simulink model "rlOvertakeTwoCars"  (R2022b)
settings: Solver=ode45  StartTime=0.0  StopTime=inf  FixedStep=0.001  RelTol=5e-3
PreLoadFcn:
  | setUpModel
PostLoadFcn:
  | setUpMain
model workspace (MAT data in the model file):
  firstWarning = 0
  originalScenarioChecksum = 'F73A6DA3C723D3CA73A6F931B7A52A9C'
values from neighbouring files (symbols this model uses):
  accel_vec = (-4:0.5:4)'    [setUpModel.m]
  amax = 3    [setUpMain.m]
  amin = -3    [setUpMain.m]
  dyNorm = [dyNorm 1.1]    [setUpSlipstream.m]
  e1_initial = 0    [setUpMain.m]
  e2_initial = 0    [setUpMain.m]
  L = data.ActorSpecifications.Length    [setUpModel.m]
  psi_o1 = 0.0058 * (pi/180)    (= 0.000101229096616)    [setUpModel.m]
  psi_o2 = 0.3528 *(pi/180)    (= 0.00615752160104)    [setUpModel.m]
  ry = [ry 0]    [setUpSlipstream.m]
  ssSwitch = 1    [setUpSlipstream.m]
  tolpsi = 10 * pi/180    (= 0.174532925199)    [setUpSlipstream.m]
  toly = 1.2*W /2    [setUpSlipstream.m]
  Ts = 0.1    [setUpMPC.m]
  TsRL = Ts    [setUpRLEnv.m]
  umax = 0.3    [setUpMain.m]
  umin = -0.3    [setUpMain.m]
  v_o1 = highSpeed1    (= 35)    [setUpModel.m]
  v_o2 = highSpeed2    (= 36)    [setUpModel.m]
  vel1 = highSpeed1 * ones(length(xlt),length(ylt))    [setUpModel.m]
  vel2 = highSpeed2 * ones(length(xlt),length(ylt))    [setUpModel.m]
  vel_vec = 0:2:20    [setUpModel.m]
  W = data.ActorSpecifications(1,1).Width    [setUpSlipstream.m]
  X_o1 = xRef1(1)    [setUpModel.m]
  X_o2 = xRef2(1)    [setUpModel.m]
  xFollow = [0 x1 xFollow 60]    [setUpSlipstream.m]
  xLead = [0 -x0 xLead]    [setUpSlipstream.m]
  xlt = -250:10:200    [setUpModel.m]
  Y_o1 = yRef1(1)    [setUpModel.m]
  Y_o2 = yRef2(1)    [setUpModel.m]
  yFollow = [c y1 yFollow 1]    [setUpSlipstream.m]
  yLead = [c y0 yLead]    [setUpSlipstream.m]
  ylt = -150:10:100    [setUpModel.m]
undefined symbols (not defined in the file or in its folder): curvature1, curvature2, deg, DiscIntNeverNeededParam, gradbp1, gradbp2, psi, rad, s, v_o, x_colpen, x_o, y_colpen, Z_colpen
libraries: simulink x26, autolibsharedcommon x22, autolibutils x10, autolibshared x10, vehdynlibtirecommon x8, drivingscenarioandsensors x4, autolibpowerinfoutils x4, sharedtransform x4, aerolibconvert2 x2, simulink_extras x2, vehdynlibtire x2, mpcadaslib x1
(part 8 of 8)

== system rlOvertakeTwoCars/Vehicle Body 3DOF Dual Track Ego/Signal Routing/Signal Routing Dual/Lateral 3DOF/Hard Point Coordinate Transform Front Left ==
  InertFrmCg : Inport
  BdyFrmCg : Inport  Port=2
  Gain : Gain  Gain=-1/2
  Hard Point Coordinate Transform External Displacement : autolibsharedcommon/Hard Point Coordinate Transform External Displacement  aMode=aMode
  Selector : Selector  InputPortWidth=2  IndexOptions=Index vector (dialog)  Indices=[1]  OutputSizes=1
  Subtract : Sum  Inputs=+-
  Vector Concatenate : Concatenate  NumInputs=3
  a : Constant  Value=a
  d : Constant  Value=d
  h : Constant  Value=h
  w : Constant  Value=w
  Inert : Outport  VectorParamsAs1DForOutWhenUnconnected=off
  Body : Outport  Port=2  VectorParamsAs1DForOutWhenUnconnected=off
  wires:
  Subtract/1 -> Vector Concatenate/2
  d/1 -> Subtract/2
  InertFrmCg/1 -> Hard Point Coordinate Transform External Displacement/1
  w/1 -> Selector/1
  Gain/1 -> Subtract/1
  a/1 -> Vector Concatenate/1
  Hard Point Coordinate Transform External Displacement/2 -> Body/1
  Vector Concatenate/1 -> Hard Point Coordinate Transform External Displacement/3
  h/1 -> Vector Concatenate/3
  BdyFrmCg/1 -> Hard Point Coordinate Transform External Displacement/2
  Hard Point Coordinate Transform External Displacement/1 -> Inert/1
  Selector/1 -> Gain/1

== system rlOvertakeTwoCars/Vehicle Body 3DOF Dual Track Ego/Signal Routing/Signal Routing Dual/Lateral 3DOF/Hard Point Coordinate Transform Front Right ==
  InertFrmCg : Inport
  BdyFrmCg : Inport  Port=2
  Gain : Gain  Gain=1/2
  Hard Point Coordinate Transform External Displacement : autolibsharedcommon/Hard Point Coordinate Transform External Displacement  aMode=aMode
  Selector : Selector  InputPortWidth=2  IndexOptions=Index vector (dialog)  Indices=[1]  OutputSizes=1
  Subtract : Sum  Inputs=+-
  Vector Concatenate : Concatenate  NumInputs=3
  a : Constant  Value=a
  d : Constant  Value=d
  h : Constant  Value=h
  w : Constant  Value=w
  Inert : Outport  VectorParamsAs1DForOutWhenUnconnected=off
  Body : Outport  Port=2  VectorParamsAs1DForOutWhenUnconnected=off
  wires:
  Subtract/1 -> Vector Concatenate/2
  a/1 -> Vector Concatenate/1
  Selector/1 -> Gain/1
  h/1 -> Vector Concatenate/3
  w/1 -> Selector/1
  d/1 -> Subtract/2
  Gain/1 -> Subtract/1
  Hard Point Coordinate Transform External Displacement/1 -> Inert/1
  BdyFrmCg/1 -> Hard Point Coordinate Transform External Displacement/2
  Vector Concatenate/1 -> Hard Point Coordinate Transform External Displacement/3
  Hard Point Coordinate Transform External Displacement/2 -> Body/1
  InertFrmCg/1 -> Hard Point Coordinate Transform External Displacement/1

== system rlOvertakeTwoCars/Vehicle Body 3DOF Dual Track Ego/Signal Routing/Signal Routing Dual/Lateral 3DOF/Hard Point Coordinate Transform Geometric ==
  InertFrmCg : Inport
  BdyFrmCg : Inport  Port=2
  Hard Point Coordinate Transform External Displacement Beta : autolibsharedcommon/Hard Point Coordinate Transform External Displacement Beta  xdot_tol=xdot_tol  aMode=aMode
  Vector Concatenate : Concatenate  NumInputs=3
  latOff : Constant  Value=latOff
  longOff : Constant  Value=longOff
  vertOff : Constant  Value=vertOff
  Inert : Outport  VectorParamsAs1DForOutWhenUnconnected=off
  Body : Outport  Port=2  VectorParamsAs1DForOutWhenUnconnected=off
  wires:
  InertFrmCg/1 -> Hard Point Coordinate Transform External Displacement Beta/1
  Hard Point Coordinate Transform External Displacement Beta/2 -> Body/1
  Vector Concatenate/1 -> Hard Point Coordinate Transform External Displacement Beta/3
  BdyFrmCg/1 -> Hard Point Coordinate Transform External Displacement Beta/2
  Hard Point Coordinate Transform External Displacement Beta/1 -> Inert/1
  vertOff/1 -> Vector Concatenate/3
  longOff/1 -> Vector Concatenate/1
  latOff/1 -> Vector Concatenate/2

== system rlOvertakeTwoCars/Vehicle Body 3DOF Dual Track Ego/Signal Routing/Signal Routing Dual/Lateral 3DOF/Hard Point Coordinate Transform Rear Left ==
  InertFrmCg : Inport
  BdyFrmCg : Inport  Port=2
  Gain : Gain  Gain=-1/2
  Hard Point Coordinate Transform External Displacement : autolibsharedcommon/Hard Point Coordinate Transform External Displacement  aMode=aMode
  Selector : Selector  InputPortWidth=2  IndexOptions=Index vector (dialog)  Indices=[2]  OutputSizes=1
  Subtract : Sum  Inputs=+-
  Vector Concatenate : Concatenate  NumInputs=3
  b : Constant  Value=-b
  d : Constant  Value=d
  h : Constant  Value=h
  w : Constant  Value=w
  Inert : Outport  VectorParamsAs1DForOutWhenUnconnected=off
  Body : Outport  Port=2  VectorParamsAs1DForOutWhenUnconnected=off
  wires:
  Gain/1 -> Subtract/1
  Subtract/1 -> Vector Concatenate/2
  w/1 -> Selector/1
  d/1 -> Subtract/2
  Selector/1 -> Gain/1
  b/1 -> Vector Concatenate/1
  h/1 -> Vector Concatenate/3
  InertFrmCg/1 -> Hard Point Coordinate Transform External Displacement/1
  Hard Point Coordinate Transform External Displacement/2 -> Body/1
  Vector Concatenate/1 -> Hard Point Coordinate Transform External Displacement/3
  BdyFrmCg/1 -> Hard Point Coordinate Transform External Displacement/2
  Hard Point Coordinate Transform External Displacement/1 -> Inert/1

== system rlOvertakeTwoCars/Vehicle Body 3DOF Dual Track Ego/Signal Routing/Signal Routing Dual/Lateral 3DOF/Hard Point Coordinate Transform Rear Right ==
  InertFrmCg : Inport
  BdyFrmCg : Inport  Port=2
  Gain : Gain  Gain=1/2
  Hard Point Coordinate Transform External Displacement : autolibsharedcommon/Hard Point Coordinate Transform External Displacement  aMode=aMode
  Selector : Selector  InputPortWidth=2  IndexOptions=Index vector (dialog)  Indices=[2]  OutputSizes=1
  Subtract : Sum  Inputs=+-
  Vector Concatenate : Concatenate  NumInputs=3
  b : Constant  Value=-b
  d : Constant  Value=d
  h : Constant  Value=h
  w : Constant  Value=w
  Inert : Outport  VectorParamsAs1DForOutWhenUnconnected=off
  Body : Outport  Port=2  VectorParamsAs1DForOutWhenUnconnected=off
  wires:
  Gain/1 -> Subtract/1
  Subtract/1 -> Vector Concatenate/2
  w/1 -> Selector/1
  d/1 -> Subtract/2
  Selector/1 -> Gain/1
  b/1 -> Vector Concatenate/1
  h/1 -> Vector Concatenate/3
  Hard Point Coordinate Transform External Displacement/1 -> Inert/1
  BdyFrmCg/1 -> Hard Point Coordinate Transform External Displacement/2
  Vector Concatenate/1 -> Hard Point Coordinate Transform External Displacement/3
  Hard Point Coordinate Transform External Displacement/2 -> Body/1
  InertFrmCg/1 -> Hard Point Coordinate Transform External Displacement/1

== system rlOvertakeTwoCars/Vehicle Body 3DOF Dual Track Ego/Signal Routing/Signal Routing Dual/Lateral 3DOF/Hitch Coordinate Transform ==
  InertFrmCg : Inport
  BodyFrmCg : Inport  Port=2
  Constant : Constant  Value=dh
  Constant1 : Constant  Value=d
  Constant2 : Constant  Value=h
  Constant3 : Constant  Value=hh
  Constant4 : Constant  Value=hl
  Hard Point Coordinate Transform External Displacement : autolibsharedcommon/Hard Point Coordinate Transform External Displacement  aMode=aMode
  Sum : Sum  Inputs=|+-
  Sum1 : Sum  Inputs=|+-
  Unary Minus2 : UnaryMinus
  Vector Concatenate : Concatenate  NumInputs=3
  Inert : Outport
  Body : Outport  Port=2
  wires:
  Constant1/1 -> Sum1/2
  Unary Minus2/1 -> Vector Concatenate/1
  Constant/1 -> Unary Minus2/1
  Sum/1 -> Vector Concatenate/3
  Constant4/1 -> Sum1/1
  Sum1/1 -> Vector Concatenate/2
  Constant3/1 -> Sum/2
  Constant2/1 -> Sum/1
  BodyFrmCg/1 -> Hard Point Coordinate Transform External Displacement/2
  InertFrmCg/1 -> Hard Point Coordinate Transform External Displacement/1
  Vector Concatenate/1 -> Hard Point Coordinate Transform External Displacement/3
  Hard Point Coordinate Transform External Displacement/1 -> Inert/1
  Hard Point Coordinate Transform External Displacement/2 -> Body/1

== system rlOvertakeTwoCars/Vehicle Body 3DOF Dual Track Ego/Signal Routing/Signal Routing Dual/Power/xdot mode ==
  note: 1) Add Subsystem or Model blocks as valid variant choices.
      | 2) You cannot connect blocks at this level. At simulation, connectivity is automatically
      | determined, based on the active variant and port name matching.
  PFExt : Inport
  PMExt : Inport  Port=2
  PFh : Inport  Port=3
  PMh : Inport  Port=4
  PFDrag : Inport  Port=5
  PFwF : Inport  Port=6
  PFwR : Inport  Port=7
  BodyFrm : Inport  Port=8
  FxIn : Subsystem  VariantControl=1
  xdotin : Subsystem  VariantControl=0
  PF : Outport  VectorParamsAs1DForOutWhenUnconnected=off
  PM : Outport  Port=2  VectorParamsAs1DForOutWhenUnconnected=off
  ax : Outport  Port=3  VectorParamsAs1DForOutWhenUnconnected=off

== system rlOvertakeTwoCars/Vehicle Body 3DOF Dual Track/Signal Routing/Signal Routing/Power/xdot mode/FxIn ==
  PFExt : Inport
  PMExt : Inport  Port=2
  PFh : Inport  Port=3
  PMh : Inport  Port=4
  PFDrag : Inport  Port=5
  PFwF : Inport  Port=6
  PFwR : Inport  Port=7
  BodyFrm : Inport  Port=8
  Bus Selector2 : BusSelector  OutputSignals=Cg.Acc.ax
  Selector1 : Selector  InputPortWidth=3  IndexOptions=Index vector (dialog)  Indices=[1 2]  OutputSizes=1
  Selector2 : Selector  InputPortWidth=3  IndexOptions=Index vector (dialog)  Indices=[3]  OutputSizes=1
  Selector3 : Selector  InputPortWidth=3  IndexOptions=Index vector (dialog)  Indices=[3]  OutputSizes=1
  Selector4 : Selector  InputPortWidth=3  IndexOptions=Index vector (dialog)  Indices=[1 2]  OutputSizes=1
  Sum : Sum  Inputs=|++
  Sum1 : Sum  Inputs=|++
  Terminator : Terminator
  Terminator2 : Terminator
  Terminator3 : Terminator
  PF : Outport  VectorParamsAs1DForOutWhenUnconnected=off
  PM : Outport  Port=2  VectorParamsAs1DForOutWhenUnconnected=off
  ax : Outport  Port=3  VectorParamsAs1DForOutWhenUnconnected=off
  wires:
  Sum1/1 -> PF/1
  Selector4/1 -> Sum1/2
  PFh/1 -> Selector4/1
  Selector2/1 -> Sum/2
  Sum/1 -> PM/1
  PMh/1 -> Selector2/1
  PFExt/1 -> Selector1/1
  PMExt/1 -> Selector3/1
  PFDrag/1 -> Terminator/1
  Selector3/1 -> Sum/1
  Selector1/1 -> Sum1/1
  PFwR/1 -> Terminator3/1
  PFwF/1 -> Terminator2/1
  BodyFrm/1 -> Bus Selector2/1
  Bus Selector2/1 -> ax/1  "<ax>"

== system rlOvertakeTwoCars/Vehicle Body 3DOF Dual Track/Signal Routing/Signal Routing/Power/xdot mode/xdotin ==
  PFExt : Inport
  PMExt : Inport  Port=2
  PFh : Inport  Port=3
  PMh : Inport  Port=4
  PFDrag : Inport  Port=5
  PFwF : Inport  Port=6
  PFwR : Inport  Port=7
  BodyFrm : Inport  Port=8
  Add : Sum  Inputs=+++++
  Ground{,1..5} (6 alike) : Ground
  Mux{,1..4} (5 alike) : Mux  Inputs=2
  Selector1 : Selector  InputPortWidth=3  IndexOptions=Index vector (dialog)  Indices=[1]  OutputSizes=1
  Selector2 : Selector  InputPortWidth=3  IndexOptions=Index vector (dialog)  Indices=[2]  OutputSizes=1
  Selector3 : Selector  InputPortWidth=3  IndexOptions=Index vector (dialog)  Indices=[3]  OutputSizes=1
  Selector4 : Selector  InputPortWidth=3  IndexOptions=Index vector (dialog)  Indices=[1]  OutputSizes=1
  Selector5 : Selector  InputPortWidth=3  IndexOptions=Index vector (dialog)  Indices=[1]  OutputSizes=1
  Selector6 : Selector  InputPortWidth=3  IndexOptions=Index vector (dialog)  Indices=[2]  OutputSizes=1
  Selector7 : Selector  InputPortWidth=3  IndexOptions=Index vector (dialog)  Indices=[3]  OutputSizes=1
  Signal Specification : SignalSpecification  Unit=gn
  Sum : Sum  Inputs=|++
  Terminator : Terminator
  Unary Minus1 : UnaryMinus
  Unary Minus2 : UnaryMinus
  Unary Minus3 : UnaryMinus
  PF : Outport  VectorParamsAs1DForOutWhenUnconnected=off
  PM : Outport  Port=2  VectorParamsAs1DForOutWhenUnconnected=off
  ax : Outport  Port=3  VectorParamsAs1DForOutWhenUnconnected=off
  wires:
  Selector7/1 -> Sum/2
  Sum/1 -> PM/1
  PMh/1 -> Selector7/1
  PFh/1 -> Selector6/1
  Mux4/1 -> Add/4
  Ground5/1 -> Mux4/1
  Selector6/1 -> Mux4/2
  Add/1 -> PF/1
  PMExt/1 -> Selector3/1
  PFExt/1 -> Selector2/1
  PFDrag/1 -> Selector1/1
  Selector1/1 -> Unary Minus3/1
  Selector2/1 -> Mux/2
  Ground/1 -> Mux/1
  Mux/1 -> Add/3
  PFwF/1 -> Selector4/1
  PFwR/1 -> Selector5/1
  Ground1/1 -> Mux2/2
  Selector4/1 -> Unary Minus1/1
  Ground2/1 -> Mux1/2
  Selector5/1 -> Unary Minus2/1
  Mux2/1 -> Add/2
  Mux1/1 -> Add/1
  Unary Minus1/1 -> Mux1/1
  Unary Minus2/1 -> Mux2/1
  Ground3/1 -> Mux3/2
  Mux3/1 -> Add/5
  Selector3/1 -> Sum/1
  Unary Minus3/1 -> Mux3/1
  BodyFrm/1 -> Terminator/1
  Ground4/1 -> Signal Specification/1
  Signal Specification/1 -> ax/1

== system rlOvertakeTwoCars/Vehicle Body 3DOF Dual Track/Signal Routing/Signal Routing/state2bus/Angle Wrap/None ==
  u : Inport
  y : Outport  VectorParamsAs1DForOutWhenUnconnected=off
  wires:
  u/1 -> y/1

== system rlOvertakeTwoCars/Vehicle Body 3DOF Dual Track/Signal Routing/Signal Routing/state2bus/xddot2ax/m^22gn ==
  ay : Inport  Unit=m/s^2
  ax : Inport  Port=2  Unit=m/s^2
  Unit Conversion : UnitConversion
  Unit Conversion1 : UnitConversion
  ay_g : Outport  Unit=gn  VectorParamsAs1DForOutWhenUnconnected=off
  ax_g : Outport  Port=2  Unit=gn  VectorParamsAs1DForOutWhenUnconnected=off
  wires:
  Unit Conversion1/1 -> ax_g/1
  Unit Conversion/1 -> ay_g/1
  ax/1 -> Unit Conversion1/1
  ay/1 -> Unit Conversion/1

== system rlOvertakeTwoCars/Vehicle Body 3DOF Dual Track/Signal Routing/Signal Routing Dual/Power/xdot mode/FxIn ==
  PFExt : Inport
  PMExt : Inport  Port=2
  PFh : Inport  Port=3
  PMh : Inport  Port=4
  PFDrag : Inport  Port=5
  PFwF : Inport  Port=6
  PFwR : Inport  Port=7
  BodyFrm : Inport  Port=8
  Bus Selector2 : BusSelector  OutputSignals=Cg.Acc.ax
  Selector1 : Selector  InputPortWidth=3  IndexOptions=Index vector (dialog)  Indices=[1 2]  OutputSizes=1
  Selector2 : Selector  InputPortWidth=3  IndexOptions=Index vector (dialog)  Indices=[3]  OutputSizes=1
  Selector3 : Selector  InputPortWidth=3  IndexOptions=Index vector (dialog)  Indices=[3]  OutputSizes=1
  Selector4 : Selector  InputPortWidth=3  IndexOptions=Index vector (dialog)  Indices=[1 2]  OutputSizes=1
  Sum : Sum  Inputs=|++
  Sum1 : Sum  Inputs=|++
  Terminator : Terminator
  Terminator2 : Terminator
  Terminator3 : Terminator
  PF : Outport  VectorParamsAs1DForOutWhenUnconnected=off
  PM : Outport  Port=2  VectorParamsAs1DForOutWhenUnconnected=off
  ax : Outport  Port=3  VectorParamsAs1DForOutWhenUnconnected=off
  wires:
  Sum1/1 -> PF/1
  Selector4/1 -> Sum1/2
  PFh/1 -> Selector4/1
  Sum/1 -> PM/1
  Selector2/1 -> Sum/2
  PMh/1 -> Selector2/1
  PFExt/1 -> Selector1/1
  PMExt/1 -> Selector3/1
  PFDrag/1 -> Terminator/1
  Selector3/1 -> Sum/1
  Selector1/1 -> Sum1/1
  PFwR/1 -> Terminator3/1
  PFwF/1 -> Terminator2/1
  BodyFrm/1 -> Bus Selector2/1
  Bus Selector2/1 -> ax/1  "<ax>"

== system rlOvertakeTwoCars/Vehicle Body 3DOF Dual Track/Signal Routing/Signal Routing Dual/Power/xdot mode/xdotin ==
  PFExt : Inport
  PMExt : Inport  Port=2
  PFh : Inport  Port=3
  PMh : Inport  Port=4
  PFDrag : Inport  Port=5
  PFwF : Inport  Port=6
  PFwR : Inport  Port=7
  BodyFrm : Inport  Port=8
  Add : Sum  Inputs=+++++
  Ground{,1..5} (6 alike) : Ground
  Mux{,1..4} (5 alike) : Mux  Inputs=2
  Selector1 : Selector  InputPortWidth=3  IndexOptions=Index vector (dialog)  Indices=[1]  OutputSizes=1
  Selector2 : Selector  InputPortWidth=3  IndexOptions=Index vector (dialog)  Indices=[2]  OutputSizes=1
  Selector3 : Selector  InputPortWidth=3  IndexOptions=Index vector (dialog)  Indices=[3]  OutputSizes=1
  Selector4 : Selector  InputPortWidth=3  IndexOptions=Index vector (dialog)  Indices=[1]  OutputSizes=1
  Selector5 : Selector  InputPortWidth=3  IndexOptions=Index vector (dialog)  Indices=[1]  OutputSizes=1
  Selector6 : Selector  InputPortWidth=3  IndexOptions=Index vector (dialog)  Indices=[3]  OutputSizes=1
  Selector7 : Selector  InputPortWidth=3  IndexOptions=Index vector (dialog)  Indices=[2]  OutputSizes=1
  Signal Specification : SignalSpecification  Unit=gn
  Sum : Sum  Inputs=|++
  Terminator : Terminator
  Unary Minus1 : UnaryMinus
  Unary Minus2 : UnaryMinus
  Unary Minus3 : UnaryMinus
  PF : Outport  VectorParamsAs1DForOutWhenUnconnected=off
  PM : Outport  Port=2  VectorParamsAs1DForOutWhenUnconnected=off
  ax : Outport  Port=3  VectorParamsAs1DForOutWhenUnconnected=off
  wires:
  Mux4/1 -> Add/4
  Ground5/1 -> Mux4/1
  Selector7/1 -> Mux4/2
  PFh/1 -> Selector7/1
  Selector6/1 -> Sum/2
  Sum/1 -> PM/1
  PMh/1 -> Selector6/1
  Add/1 -> PF/1
  PMExt/1 -> Selector3/1
  PFExt/1 -> Selector2/1
  PFDrag/1 -> Selector1/1
  Selector1/1 -> Unary Minus3/1
  Selector2/1 -> Mux/2
  Ground/1 -> Mux/1
  Mux/1 -> Add/3
  PFwF/1 -> Selector4/1
  PFwR/1 -> Selector5/1
  Ground1/1 -> Mux2/2
  Selector4/1 -> Unary Minus1/1
  Ground2/1 -> Mux1/2
  Selector5/1 -> Unary Minus2/1
  Mux2/1 -> Add/2
  Mux1/1 -> Add/1
  Unary Minus1/1 -> Mux1/1
  Unary Minus2/1 -> Mux2/1
  Ground3/1 -> Mux3/2
  Mux3/1 -> Add/5
  Selector3/1 -> Sum/1
  Unary Minus3/1 -> Mux3/1
  BodyFrm/1 -> Terminator/1
  Ground4/1 -> Signal Specification/1
  Signal Specification/1 -> ax/1

== system rlOvertakeTwoCars/Vehicle Body 3DOF Dual Track Ego/Signal Routing/Signal Routing/Power/xdot mode/FxIn ==
  PFExt : Inport
  PMExt : Inport  Port=2
  PFh : Inport  Port=3
  PMh : Inport  Port=4
  PFDrag : Inport  Port=5
  PFwF : Inport  Port=6
  PFwR : Inport  Port=7
  BodyFrm : Inport  Port=8
  Bus Selector2 : BusSelector  OutputSignals=Cg.Acc.ax
  Selector1 : Selector  InputPortWidth=3  IndexOptions=Index vector (dialog)  Indices=[1 2]  OutputSizes=1
  Selector2 : Selector  InputPortWidth=3  IndexOptions=Index vector (dialog)  Indices=[3]  OutputSizes=1
  Selector3 : Selector  InputPortWidth=3  IndexOptions=Index vector (dialog)  Indices=[3]  OutputSizes=1
  Selector4 : Selector  InputPortWidth=3  IndexOptions=Index vector (dialog)  Indices=[1 2]  OutputSizes=1
  Sum : Sum  Inputs=|++
  Sum1 : Sum  Inputs=|++
  Terminator : Terminator
  Terminator2 : Terminator
  Terminator3 : Terminator
  PF : Outport  VectorParamsAs1DForOutWhenUnconnected=off
  PM : Outport  Port=2  VectorParamsAs1DForOutWhenUnconnected=off
  ax : Outport  Port=3  VectorParamsAs1DForOutWhenUnconnected=off
  wires:
  Sum1/1 -> PF/1
  Selector4/1 -> Sum1/2
  PFh/1 -> Selector4/1
  Selector2/1 -> Sum/2
  Sum/1 -> PM/1
  PMh/1 -> Selector2/1
  PFExt/1 -> Selector1/1
  PMExt/1 -> Selector3/1
  PFDrag/1 -> Terminator/1
  Selector3/1 -> Sum/1
  Selector1/1 -> Sum1/1
  PFwR/1 -> Terminator3/1
  PFwF/1 -> Terminator2/1
  BodyFrm/1 -> Bus Selector2/1
  Bus Selector2/1 -> ax/1  "<ax>"

== system rlOvertakeTwoCars/Vehicle Body 3DOF Dual Track Ego/Signal Routing/Signal Routing/Power/xdot mode/xdotin ==
  PFExt : Inport
  PMExt : Inport  Port=2
  PFh : Inport  Port=3
  PMh : Inport  Port=4
  PFDrag : Inport  Port=5
  PFwF : Inport  Port=6
  PFwR : Inport  Port=7
  BodyFrm : Inport  Port=8
  Add : Sum  Inputs=+++++
  Ground{,1..5} (6 alike) : Ground
  Mux{,1..4} (5 alike) : Mux  Inputs=2
  Selector1 : Selector  InputPortWidth=3  IndexOptions=Index vector (dialog)  Indices=[1]  OutputSizes=1
  Selector2 : Selector  InputPortWidth=3  IndexOptions=Index vector (dialog)  Indices=[2]  OutputSizes=1
  Selector3 : Selector  InputPortWidth=3  IndexOptions=Index vector (dialog)  Indices=[3]  OutputSizes=1
  Selector4 : Selector  InputPortWidth=3  IndexOptions=Index vector (dialog)  Indices=[1]  OutputSizes=1
  Selector5 : Selector  InputPortWidth=3  IndexOptions=Index vector (dialog)  Indices=[1]  OutputSizes=1
  Selector6 : Selector  InputPortWidth=3  IndexOptions=Index vector (dialog)  Indices=[2]  OutputSizes=1
  Selector7 : Selector  InputPortWidth=3  IndexOptions=Index vector (dialog)  Indices=[3]  OutputSizes=1
  Signal Specification : SignalSpecification  Unit=gn
  Sum : Sum  Inputs=|++
  Terminator : Terminator
  Unary Minus1 : UnaryMinus
  Unary Minus2 : UnaryMinus
  Unary Minus3 : UnaryMinus
  PF : Outport  VectorParamsAs1DForOutWhenUnconnected=off
  PM : Outport  Port=2  VectorParamsAs1DForOutWhenUnconnected=off
  ax : Outport  Port=3  VectorParamsAs1DForOutWhenUnconnected=off
  wires:
  Selector7/1 -> Sum/2
  Sum/1 -> PM/1
  PMh/1 -> Selector7/1
  PFh/1 -> Selector6/1
  Mux4/1 -> Add/4
  Ground5/1 -> Mux4/1
  Selector6/1 -> Mux4/2
  Add/1 -> PF/1
  PMExt/1 -> Selector3/1
  PFExt/1 -> Selector2/1
  PFDrag/1 -> Selector1/1
  Selector1/1 -> Unary Minus3/1
  Selector2/1 -> Mux/2
  Ground/1 -> Mux/1
  Mux/1 -> Add/3
  PFwF/1 -> Selector4/1
  PFwR/1 -> Selector5/1
  Ground1/1 -> Mux2/2
  Selector4/1 -> Unary Minus1/1
  Ground2/1 -> Mux1/2
  Selector5/1 -> Unary Minus2/1
  Mux2/1 -> Add/2
  Mux1/1 -> Add/1
  Unary Minus1/1 -> Mux1/1
  Unary Minus2/1 -> Mux2/1
  Ground3/1 -> Mux3/2
  Mux3/1 -> Add/5
  Selector3/1 -> Sum/1
  Unary Minus3/1 -> Mux3/1
  BodyFrm/1 -> Terminator/1
  Ground4/1 -> Signal Specification/1
  Signal Specification/1 -> ax/1

== system rlOvertakeTwoCars/Vehicle Body 3DOF Dual Track Ego/Signal Routing/Signal Routing/state2bus/Angle Wrap/None ==
  u : Inport
  y : Outport  VectorParamsAs1DForOutWhenUnconnected=off
  wires:
  u/1 -> y/1

== system rlOvertakeTwoCars/Vehicle Body 3DOF Dual Track Ego/Signal Routing/Signal Routing/state2bus/xddot2ax/m^22gn ==
  ay : Inport  Unit=m/s^2
  ax : Inport  Port=2  Unit=m/s^2
  Unit Conversion : UnitConversion
  Unit Conversion1 : UnitConversion
  ay_g : Outport  Unit=gn  VectorParamsAs1DForOutWhenUnconnected=off
  ax_g : Outport  Port=2  Unit=gn  VectorParamsAs1DForOutWhenUnconnected=off
  wires:
  Unit Conversion1/1 -> ax_g/1
  Unit Conversion/1 -> ay_g/1
  ax/1 -> Unit Conversion1/1
  ay/1 -> Unit Conversion/1

== system rlOvertakeTwoCars/Vehicle Body 3DOF Dual Track Ego/Signal Routing/Signal Routing Dual/Power/xdot mode/FxIn ==
  PFExt : Inport
  PMExt : Inport  Port=2
  PFh : Inport  Port=3
  PMh : Inport  Port=4
  PFDrag : Inport  Port=5
  PFwF : Inport  Port=6
  PFwR : Inport  Port=7
  BodyFrm : Inport  Port=8
  Bus Selector2 : BusSelector  OutputSignals=Cg.Acc.ax
  Selector1 : Selector  InputPortWidth=3  IndexOptions=Index vector (dialog)  Indices=[1 2]  OutputSizes=1
  Selector2 : Selector  InputPortWidth=3  IndexOptions=Index vector (dialog)  Indices=[3]  OutputSizes=1
  Selector3 : Selector  InputPortWidth=3  IndexOptions=Index vector (dialog)  Indices=[3]  OutputSizes=1
  Selector4 : Selector  InputPortWidth=3  IndexOptions=Index vector (dialog)  Indices=[1 2]  OutputSizes=1
  Sum : Sum  Inputs=|++
  Sum1 : Sum  Inputs=|++
  Terminator : Terminator
  Terminator2 : Terminator
  Terminator3 : Terminator
  PF : Outport  VectorParamsAs1DForOutWhenUnconnected=off
  PM : Outport  Port=2  VectorParamsAs1DForOutWhenUnconnected=off
  ax : Outport  Port=3  VectorParamsAs1DForOutWhenUnconnected=off
  wires:
  Sum1/1 -> PF/1
  Selector4/1 -> Sum1/2
  PFh/1 -> Selector4/1
  Sum/1 -> PM/1
  Selector2/1 -> Sum/2
  PMh/1 -> Selector2/1
  PFExt/1 -> Selector1/1
  PMExt/1 -> Selector3/1
  PFDrag/1 -> Terminator/1
  Selector3/1 -> Sum/1
  Selector1/1 -> Sum1/1
  PFwR/1 -> Terminator3/1
  PFwF/1 -> Terminator2/1
  BodyFrm/1 -> Bus Selector2/1
  Bus Selector2/1 -> ax/1  "<ax>"

== system rlOvertakeTwoCars/Vehicle Body 3DOF Dual Track Ego/Signal Routing/Signal Routing Dual/Power/xdot mode/xdotin ==
  PFExt : Inport
  PMExt : Inport  Port=2
  PFh : Inport  Port=3
  PMh : Inport  Port=4
  PFDrag : Inport  Port=5
  PFwF : Inport  Port=6
  PFwR : Inport  Port=7
  BodyFrm : Inport  Port=8
  Add : Sum  Inputs=+++++
  Ground{,1..5} (6 alike) : Ground
  Mux{,1..4} (5 alike) : Mux  Inputs=2
  Selector1 : Selector  InputPortWidth=3  IndexOptions=Index vector (dialog)  Indices=[1]  OutputSizes=1
  Selector2 : Selector  InputPortWidth=3  IndexOptions=Index vector (dialog)  Indices=[2]  OutputSizes=1
  Selector3 : Selector  InputPortWidth=3  IndexOptions=Index vector (dialog)  Indices=[3]  OutputSizes=1
  Selector4 : Selector  InputPortWidth=3  IndexOptions=Index vector (dialog)  Indices=[1]  OutputSizes=1
  Selector5 : Selector  InputPortWidth=3  IndexOptions=Index vector (dialog)  Indices=[1]  OutputSizes=1
  Selector6 : Selector  InputPortWidth=3  IndexOptions=Index vector (dialog)  Indices=[3]  OutputSizes=1
  Selector7 : Selector  InputPortWidth=3  IndexOptions=Index vector (dialog)  Indices=[2]  OutputSizes=1
  Signal Specification : SignalSpecification  Unit=gn
  Sum : Sum  Inputs=|++
  Terminator : Terminator
  Unary Minus1 : UnaryMinus
  Unary Minus2 : UnaryMinus
  Unary Minus3 : UnaryMinus
  PF : Outport  VectorParamsAs1DForOutWhenUnconnected=off
  PM : Outport  Port=2  VectorParamsAs1DForOutWhenUnconnected=off
  ax : Outport  Port=3  VectorParamsAs1DForOutWhenUnconnected=off
  wires:
  Mux4/1 -> Add/4
  Ground5/1 -> Mux4/1
  Selector7/1 -> Mux4/2
  PFh/1 -> Selector7/1
  Selector6/1 -> Sum/2
  Sum/1 -> PM/1
  PMh/1 -> Selector6/1
  Add/1 -> PF/1
  PMExt/1 -> Selector3/1
  PFExt/1 -> Selector2/1
  PFDrag/1 -> Selector1/1
  Selector1/1 -> Unary Minus3/1
  Selector2/1 -> Mux/2
  Ground/1 -> Mux/1
  Mux/1 -> Add/3
  PFwF/1 -> Selector4/1
  PFwR/1 -> Selector5/1
  Ground1/1 -> Mux2/2
  Selector4/1 -> Unary Minus1/1
  Ground2/1 -> Mux1/2
  Selector5/1 -> Unary Minus2/1
  Mux2/1 -> Add/2
  Mux1/1 -> Add/1
  Unary Minus1/1 -> Mux1/1
  Unary Minus2/1 -> Mux2/1
  Ground3/1 -> Mux3/2
  Mux3/1 -> Add/5
  Selector3/1 -> Sum/1
  Unary Minus3/1 -> Mux3/1
  BodyFrm/1 -> Terminator/1
  Ground4/1 -> Signal Specification/1
  Signal Specification/1 -> ax/1

== matlab function rlOvertakeTwoCars/Vehicle Body 3DOF Dual Track Ego/Signal Routing/Signal Routing/state2bus/COMB2I ==
  data: x input size=4; y output size=2
function y = fcn(x)%#codegen
coder.allowpcode('plain')
y = automlvehb2i(x);

== matlab function rlOvertakeTwoCars/Final Trajectory Bird's-Eye Visualization Lead/MATLAB Function ==
  data: pos input; egoActor output Bus: BusActorsActors; vel input; yaw input; yawRate input
function egoActor = packEgo(pos,vel,yaw,yawRate)
% Pack ego information into a single ego actor bus
%
% Imoprtant note:
% Output is a bus of type BusActorsActors. This is the same bus used by the
% Scenario Reader to output an individual actor. If you change the
% output bus name of Scenario Reader, change the output bus name here
% as well by clicking on 'Edit Data' in the menu above.

egoActor = struct(...
    'ActorID',1,...
    'Position', [pos(1) pos(2) 0], ...
    'Velocity', [vel(1) vel(2) 0], ...
    'Roll', 0, ...
    'Pitch', 0, ...
    'Yaw', yaw, ...
    'AngularVelocity', [0 0 yawRate]);

== matlab function rlOvertakeTwoCars/Vehicle Body 3DOF Dual Track Ego/Signal Routing/Signal Routing Dual/state2bus/COMB2I ==
  data: x input size=4; y output size=2
function y = fcn(x)%#codegen
coder.allowpcode('plain')
y = automlvehb2i(x);

== matlab function rlOvertakeTwoCars/Vehicle Body 3DOF Dual Track Ego/vehicle model ==
  data: delta_f input; delta_r input; mu input; a parameter; b parameter; h parameter; d parameter; w parameter; m parameter; NF parameter; NR parameter; Izz parameter; g parameter; Fxtire_sat parameter size=1; Fytire_sat parameter size=1; trackMode parameter; inputMode parameter; xdot_tol parameter; Fznom parameter size=1; F_f input; F_r input; F_ext input size=3; M_ext input size=3; Fh input size=3; Mh input size=3; Cy_f input; Cy_r input; dh input; hl input; hh input; yOut output size=3; FBody output size=3; MBody output size=3; FOut output; FTire output; Fg output size=3; wheelInfo output; stateDer output size=4; stateVec input size=4; status output size=1
function [yOut,FBody,MBody,FOut,FTire,Fg,wheelInfo,stateDer,status] = fcn(delta_f,delta_r,mu,a,b,h,d,w,m,NF,NR,Izz,g,Fxtire_sat,Fytire_sat,trackMode,inputMode,xdot_tol,Fznom,F_f,F_r,F_ext,M_ext,Fh,Mh,Cy_f,Cy_r,dh,hl,hh,stateVec)%#codegen
coder.allowpcode('plain')
switch trackMode
    case 1
       [yOut,FBody,MBody,FOut,FTire,Fg,wheelInfo,stateDer,status] = automlvehdynbicycle(delta_f,delta_r,mu,a,b,h,m,NF,NR,Izz,g,Fxtire_sat,Fytire_sat,inputMode,xdot_tol,Fznom,F_f,F_r,F_ext,M_ext,Fh,Mh,Cy_f,Cy_r,dh,hh,stateVec);
    case 2
       [yOut,FBody,MBody,FOut,FTire,Fg,wheelInfo,stateDer,status] = automlvehdyndualtrack(delta_f,delta_r,mu,a,b,h,d,w,m,NF,NR,Izz,g,Fxtire_sat,Fytire_sat,inputMode,xdot_tol,Fznom,F_f,F_r,F_ext,M_ext,Fh,Mh,Cy_f,Cy_r,dh,hl,hh,stateVec);
end
end

== matlab function rlOvertakeTwoCars/Final Trajectory Bird's-Eye Visualization Ego/MATLAB Function ==
  data: pos input; egoActor output Bus: BusActorsActors; vel input; yaw input; yawRate input
function egoActor = packEgo(pos,vel,yaw,yawRate)
% Pack ego information into a single ego actor bus
%
% Imoprtant note:
% Output is a bus of type BusActorsActors. This is the same bus used by the
% Scenario Reader to output an individual actor. If you change the
% output bus name of Scenario Reader, change the output bus name here
% as well by clicking on 'Edit Data' in the menu above.

egoActor = struct(...
    'ActorID',2,...
    'Position', [pos(1) pos(2) 0], ...
    'Velocity', [vel(1) vel(2) 0], ...
    'Roll', 0, ...
    'Pitch', 0, ...
    'Yaw', yaw, ...
    'AngularVelocity', [0 0 yawRate]);

== matlab function rlOvertakeTwoCars/Vehicle Body 3DOF Dual Track/Signal Routing/Signal Routing Dual/state2bus/COMB2I ==
  data: x input size=4; y output size=2
function y = fcn(x)%#codegen
coder.allowpcode('plain')
y = automlvehb2i(x);

== matlab function rlOvertakeTwoCars/Vehicle Body 3DOF Dual Track/Signal Routing/Signal Routing/state2bus/COMB2I ==
  data: x input size=4; y output size=2
function y = fcn(x)%#codegen
coder.allowpcode('plain')
y = automlvehb2i(x);

== matlab function rlOvertakeTwoCars/Vehicle Body 3DOF Dual Track/vehicle model ==
  data: delta_f input; delta_r input; mu input; a parameter; b parameter; h parameter; d parameter; w parameter; m parameter; NF parameter; NR parameter; Izz parameter; g parameter; Fxtire_sat parameter size=1; Fytire_sat parameter size=1; trackMode parameter; inputMode parameter; xdot_tol parameter; Fznom parameter size=1; F_f input; F_r input; F_ext input size=3; M_ext input size=3; Fh input size=3; Mh input size=3; Cy_f input; Cy_r input; dh input; hl input; hh input; yOut output size=3; FBody output size=3; MBody output size=3; FOut output; FTire output; Fg output size=3; wheelInfo output; stateDer output size=4; stateVec input size=4; status output size=1
function [yOut,FBody,MBody,FOut,FTire,Fg,wheelInfo,stateDer,status] = fcn(delta_f,delta_r,mu,a,b,h,d,w,m,NF,NR,Izz,g,Fxtire_sat,Fytire_sat,trackMode,inputMode,xdot_tol,Fznom,F_f,F_r,F_ext,M_ext,Fh,Mh,Cy_f,Cy_r,dh,hl,hh,stateVec)%#codegen
coder.allowpcode('plain')
switch trackMode
    case 1
       [yOut,FBody,MBody,FOut,FTire,Fg,wheelInfo,stateDer,status] = automlvehdynbicycle(delta_f,delta_r,mu,a,b,h,m,NF,NR,Izz,g,Fxtire_sat,Fytire_sat,inputMode,xdot_tol,Fznom,F_f,F_r,F_ext,M_ext,Fh,Mh,Cy_f,Cy_r,dh,hh,stateVec);
    case 2
       [yOut,FBody,MBody,FOut,FTire,Fg,wheelInfo,stateDer,status] = automlvehdyndualtrack(delta_f,delta_r,mu,a,b,h,d,w,m,NF,NR,Izz,g,Fxtire_sat,Fytire_sat,inputMode,xdot_tol,Fznom,F_f,F_r,F_ext,M_ext,Fh,Mh,Cy_f,Cy_r,dh,hl,hh,stateVec);
end
end
